simulink model "MKR_1000_IMU_Matlab"  (R2022b)
settings: Solver=VariableStepAuto  StartTime=0.0  StopTime=10.0  RelTol=1e-3  EnableMultiTasking=on
libraries: arduinosensorlib x1
settings Model: ExtModeTrigDuration=2  Creator=xavier.pessoles2  LastModifiedBy=xavier.pessoles2
settings RTWCC: BuildConfiguration=Faster Runs

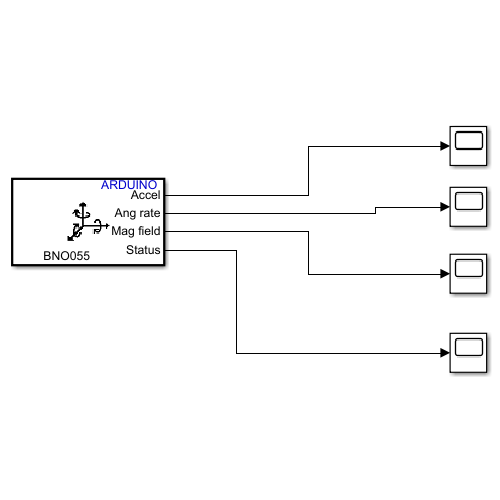
[thumbnail: Simulink's stored preview of the top-level diagram]
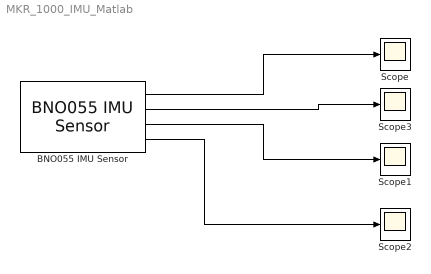
== system MKR_1000_IMU_Matlab ==
  BNO055 IMU Sensor : arduinosensorlib/BNO055 IMU Sensor  SlaveAddress=0x28  OperationMode=Fusion  Accel=on  AngularRate=on  MagField=on  EulerAngles=off  Quat=off  LinearAccel=off  GravityVector=off  Status=on  Timestamp=off  AccelRange=4G  AccelBW=62.5 Hz  GyroRange=2000 dps  GyroBW=32 Hz  MagODR=10 Hz  spf=1  SampleTime=-1  blockPlatform=ARDUINO  QueueSizeFactor=1
  Scope{,1..3} (4 alike) : Scope
  wires:
  BNO055 IMU Sensor/1 -> Scope/1
  BNO055 IMU Sensor/3 -> Scope1/1
  BNO055 IMU Sensor/4 -> Scope2/1
  BNO055 IMU Sensor/2 -> Scope3/1
